simulink model "Collect2a_Model"  (R2024b)
settings: Solver=VariableStepAuto  StartTime=0.0  StopTime=10.0  RelTol=1e-3
libraries: NSA_DEVS_SINKS x3, NSA_DEVS_LOGISTICS x2, NSA_DEVS_SOURCES x2, NSA_DEVS_ROUTING x1
settings Model: Creator=david  LastModifiedBy=peter
settings RTWCC: GPUComputeCapability=3.5

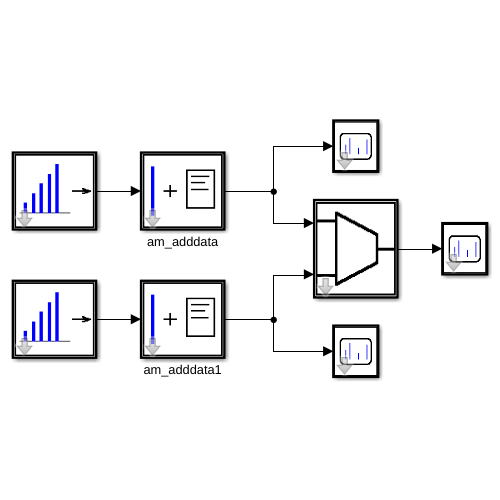
[thumbnail: Simulink's stored preview of the top-level diagram]
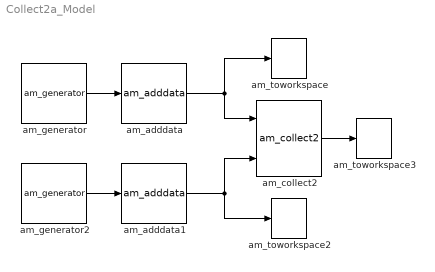
== system Collect2a_Model ==
  am_adddata : NSA_DEVS_LOGISTICS/am_adddata  fields="[\"name\"]"  values="[\"Peter\"]"  numeric=[false]  infield="\"id\""  tau=[0,1]  debug=0
      settings: SourceProductName=Logistics
  am_adddata1 : NSA_DEVS_LOGISTICS/am_adddata  fields="[\"name\"]"  values="[\"Peter\"]"  numeric=[false]  infield="\"id\""  tau=[0,1]  debug=0
      settings: SourceProductName=Logistics
  am_collect2 : NSA_DEVS_ROUTING/am_collect2  tD=[0,2]  tau=[0,1]  debug=0
      settings: SourceProductName=Routing
  am_generator : NSA_DEVS_SOURCES/am_generator  tG=1  n0=1  nG=10  tD=[0,2]  debug=0
      settings: SourceProductName=Sources
  am_generator2 : NSA_DEVS_SOURCES/am_generator  tG=2.5  n0=11  nG=10  tD=[0,2]  debug=0
      settings: SourceProductName=Sources
  am_toworkspace : NSA_DEVS_SINKS/am_toworkspace  varname="\"gen1Out\""  t0=0  format="\"vector\""  tau=[0,1]  debug=0
      settings: SourceProductName=Sinks
  am_toworkspace2 : NSA_DEVS_SINKS/am_toworkspace  varname="\"gen2Out\""  t0=0  format="\"vector\""  tau=[0,1]  debug=0
      settings: SourceProductName=Sinks
  am_toworkspace3 : NSA_DEVS_SINKS/am_toworkspace  varname="\"combOut\""  t0=0  format="\"vector\""  tau=[0,1]  debug=0
      settings: SourceProductName=Sinks
  wires:
  am_generator/1 -> am_adddata/1
  am_generator2/1 -> am_adddata1/1
  am_collect2/1 -> am_toworkspace3/1
  am_adddata/1 -> am_toworkspace/1, am_collect2/1
  am_adddata1/1 -> am_toworkspace2/1, am_collect2/2
